simulink model "Bias_estimation_KF"  (R2018b)
settings: Solver=FixedStepDiscrete  StartTime=0.0  StopTime=SIM_TIME  RelTol=1e-3
values from neighbouring files (symbols this model uses):
  C = [1 0]    [Bias_estimation.m]
  Ts = 0.01    [Bias_estimation.m]
  xhat0 = zeros(2,1)    [Bias_estimation.m]
undefined symbols (not defined in the file or in its folder): F, G, Ld1
settings Model: Creator=Roberto  LastModifiedBy=Roberto
settings SFSimCC: SimUseLocalCustomCode=off
settings RTWCC: RTWUseLocalCustomCode=off

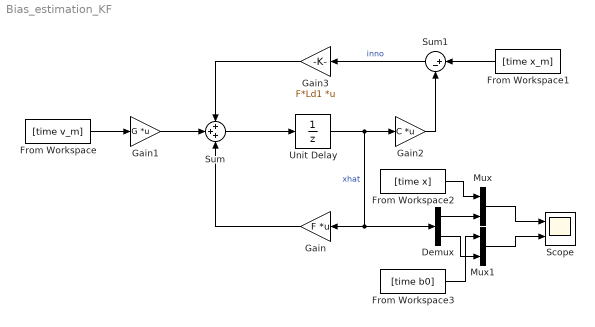
== system Bias_estimation_KF ==
  Demux : Demux  Outputs=2
  From Workspace : FromWorkspace  VariableName=[time v_m]  SampleTime=Ts  OutputAfterFinalValue=Setting to zero
  From Workspace1 : FromWorkspace  VariableName=[time x_m]  SampleTime=Ts  OutputAfterFinalValue=Setting to zero
  From Workspace2 : FromWorkspace  VariableName=[time x]  SampleTime=Ts  OutputAfterFinalValue=Setting to zero
  From Workspace3 : FromWorkspace  VariableName=[time b0]  SampleTime=Ts  OutputAfterFinalValue=Setting to zero
  Gain : Gain  Gain=F  Multiplication=Matrix(K*u) (u vector)
  Gain1 : Gain  Gain=G  Multiplication=Matrix(K*u) (u vector)
  Gain2 : Gain  Gain=C  Multiplication=Matrix(K*u) (u vector)
  Gain3 : Gain  Gain=F*Ld1  Multiplication=Matrix(K*u) (u vector)
  Mux : Mux  Inputs=2
  Mux1 : Mux  Inputs=2
  Scope : Scope  NumInputPorts=2
  Sum : Sum  Inputs=+++
  Sum1 : Sum  Inputs=|+-
  Unit Delay : UnitDelay  InitialCondition=xhat0  SampleTime=Ts
  wires:
  From Workspace/1 -> Gain1/1
  Gain/1 -> Sum/3
  Sum/1 -> Unit Delay/1
  Gain1/1 -> Sum/2
  Unit Delay/1 -> Demux/1, Gain/1, Gain2/1  "xhat"
  Gain3/1 -> Sum/1
  From Workspace1/1 -> Sum1/1
  Gain2/1 -> Sum1/2
  Sum1/1 -> Gain3/1  "inno"
  Demux/1 -> Mux/2
  Mux/1 -> Scope/1
  From Workspace2/1 -> Mux/1
  Demux/2 -> Mux1/2
  From Workspace3/1 -> Mux1/1
  Mux1/1 -> Scope/2
